simulink model "ConvertTo_BFloat16_Ex1"  (R2024a)
settings: Solver=VariableStepAuto  StartTime=0.0  StopTime=1  RelTol=1e-3
undefined symbols (not defined in the file): AIE, i, L, ML, nsvh1369, xcvc2602
libraries: aieUtilities x1, vmcUtilities x1, dspsrcs4 x1
settings Model: Creator=sdegala  LastModifiedBy=robg
settings RTWCC: GPUComputeCapability=3.5
settings ConfigComp: CovBoundaryAbsTol=1.0e-5

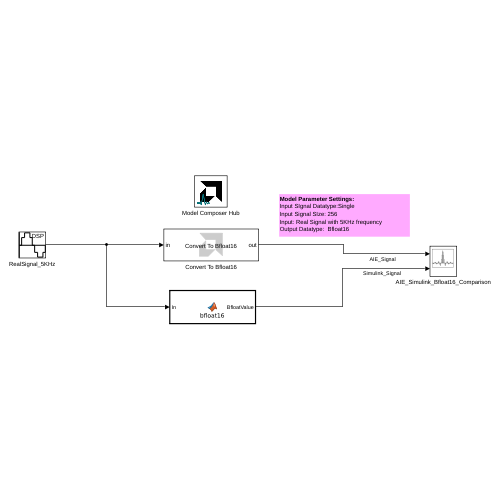
[thumbnail: Simulink's stored preview of the top-level diagram]
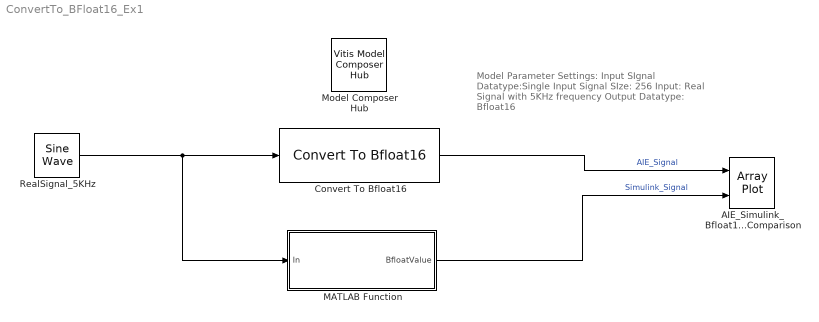
== system ConvertTo_BFloat16_Ex1 ==
  note: Model Parameter Settings:
      | Input SIgnal Datatype:Single
      | Input Signal SIze: 256
      | Input: Real Signal with 5KHz frequency
      | Output Datatype: Bfloat16
  AIE_Simulink_Bfloat16_Comparison : ArrayPlot  NumInputPorts=2  WindowPosition=[1.000000,6.000000,1274.000000,655.000000,]  Visible=on  ScopeFrameLocation=window  PlotType=Line  YLimits=[-1.25,1.25]  ShowLegend=on  DefaultConfigurationName=dsp.scopes.ArrayPlotBlockSpecification
  Convert To Bfloat16 : aieUtilities/Convert To Bfloat16
  MATLAB Function : MATLAB Function  TreatAsAtomicUnit=on
  Model Composer Hub : vmcUtilities/Vitis Model Composer Hub  Tag=genX  CodeGeneration=off  SubsystemName=AIE_FFT_Subsystem  StartColumn=1  NumberOfColumns=1  TargetDirectory=./code  exportDesign=off  analyzeDesign=off  validateDesignOnHw=off  ExportType=AI Engines  IpVendor=xilinx.com  IpLibrary=hls  IpVersion=1.0  IpHWLanguage=Verilog  AieCompilerOptions={}  AieSimulatorOptions={}  CreateTestbench=on  TestbenchStackSize=10  RunRtlSim=off  RunCSim=off  RunAieSim=on  AieSimTimeout=50000  RunAieSimProfiling=off  LaunchVitisAnalyzer=off  PlotOutput=off  RunX86Sim=off  X86SimTimeout=10  GenHwImage=off  GenLibadfXo=off  GenHwValidationCode=off  PlatformType=Not Specified  HwSystemType=Baremetal  HwValidationTarget=hw  ProjDevice=xcvc2602-nsvh1369-1LHP-i-L  ProjDevicePart=xcvc2602-nsvh1369-1LHP-i-L  AIEType=AIE-ML  SamplePeriod=-1  ClockFrequency=200  DataPathParallelism=1  xilinxfamily=versalaicore  part=xcvc2602  speed=-1LHP-i-L  package=nsvh1369  directory=./netlist  testbench=off  incr_netlist=off  synthesis_tool=Vivado  clock_wrapper=Clock Enables  dbl_ovrd=According to Block Masks  dcm_input_clock_period=10  sysclk_period=10  simulink_period=1  eval_field=0  LogFileName=/proj/xcoswmktg/robg/git/vmc_examples/gitent/Examples/AIENGINE/DSPlib/Dynamic_FFT/code/model_composer.log  NThreads=4
  RealSignal_5KHz : dspsrcs4/Sine Wave  Amplitude=1  Frequency=5e3  Phase=0  SampleMode=Discrete  OutComplex=Real  CompMethod=Trigonometric fcn  TableSize=Speed  SampleTime=1/20e3  SamplesPerFrame=256  ResetState=Restart at time zero  OutputFrames=off  dataType=single  wordLen=16  udDataType=sfix(16)  fracBitsMode=User-defined  numFracBits=0  OutDataTypeStr=single  LastOutDataTypeStr=single
  wires:
  RealSignal_5KHz/1 -> MATLAB Function/1(In), Convert To Bfloat16/1
  Convert To Bfloat16/1 -> AIE_Simulink_Bfloat16_Comparison/1  "AIE_Signal"
  MATLAB Function/1(BfloatValue) -> AIE_Simulink_Bfloat16_Comparison/2  "Simulink_Signal"

== matlab function ConvertTo_BFloat16_Ex1/MATLAB Function ==
  data: In input; BfloatValue output
function  BfloatValue = bfloat16(In)

Bfloat16 = CustomFloat(In, 16, 7); 
BfloatValue = single(Bfloat16);

% Fraction: 7 bits
% Exponent: 8 bits
